simulink model "modello_nave"  (R2023b)
settings: Solver=VariableStepAuto  StartTime=0.0  StopTime=10.0  RelTol=1e-3
values from neighbouring files (symbols this model uses):
  Km1 = 1    [prova_matrici.m]
  Km2 = 1    [prova_matrici.m]
  phi_0 = 0    [prova_matrici.m]
  r_0 = 0    [prova_matrici.m]
  T1 = 1    [prova_matrici.m]
  Tm1 = 1    [prova_matrici.m]
  Tm2 = 1    [prova_matrici.m]
  u_0 = 0    [prova_matrici.m]
  v_0 = 0    [prova_matrici.m]
settings Model: Creator=edoca  LastModifiedBy=jacoc

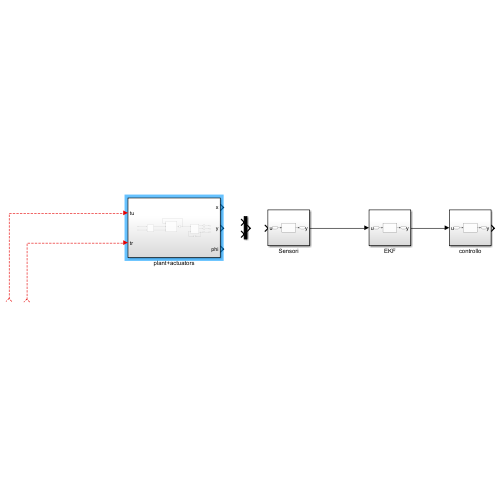
[thumbnail: Simulink's stored preview of the top-level diagram]
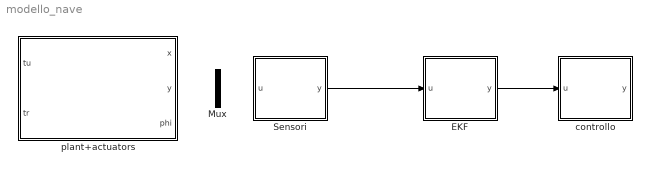
== system modello_nave ==
  EKF : Subsystem
  Mux : Mux  Inputs=2
  Sensori : Subsystem
  controllo : Subsystem
  plant+actuators : Subsystem
  wires:
  ? -> plant+actuators/1(tu)
  ? -> plant+actuators/2(tr)
  EKF/1(y) -> controllo/1(u)
  Sensori/1(y) -> EKF/1(u)

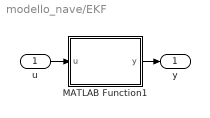
== system modello_nave/EKF ==
  u : Inport
  MATLAB Function1 : MATLAB Function  TreatAsAtomicUnit=on
  y : Outport
  wires:
  u/1 -> MATLAB Function1/1(u)
  MATLAB Function1/1(y) -> y/1

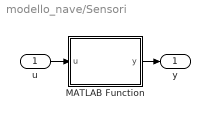
== system modello_nave/Sensori ==
  u : Inport
  MATLAB Function : MATLAB Function  TreatAsAtomicUnit=on
  y : Outport
  wires:
  u/1 -> MATLAB Function/1(u)
  MATLAB Function/1(y) -> y/1

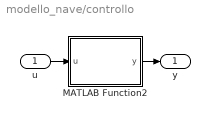
== system modello_nave/controllo ==
  u : Inport
  MATLAB Function2 : MATLAB Function  TreatAsAtomicUnit=on
  y : Outport
  wires:
  u/1 -> MATLAB Function2/1(u)
  MATLAB Function2/1(y) -> y/1

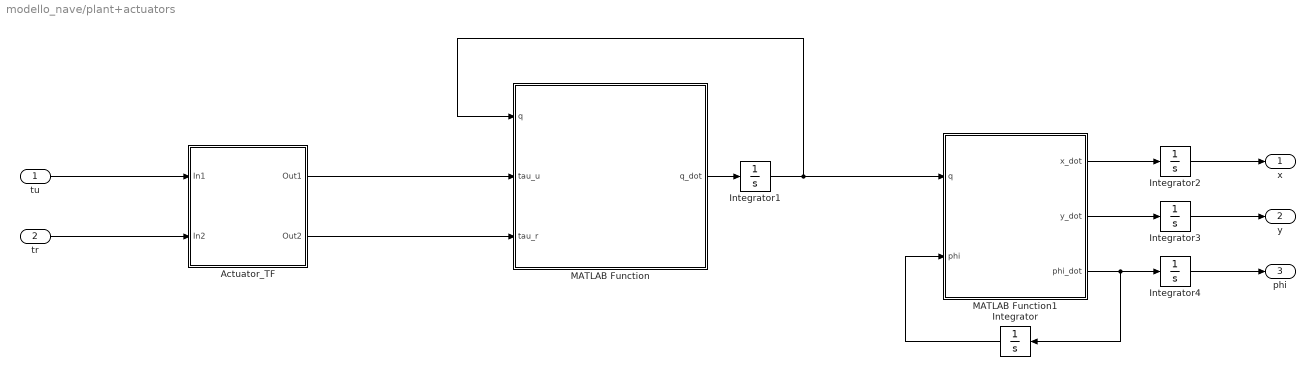
== system modello_nave/plant+actuators ==
  tu : Inport
  tr : Inport  Port=2
  Actuator_TF : Subsystem
  Integrator{,2..4} (4 alike) : Integrator  InitialCondition=phi_0
  Integrator1 : Integrator  InitialCondition=[u_0; v_0; r_0]
  MATLAB Function : MATLAB Function  TreatAsAtomicUnit=on
  MATLAB Function1 : MATLAB Function  TreatAsAtomicUnit=on
  x : Outport
  y : Outport  Port=2
  phi : Outport  Port=3
  wires:
  Integrator1/1 -> MATLAB Function/1(q), MATLAB Function1/1(q)
  MATLAB Function/1(q_dot) -> Integrator1/1
  Integrator/1 -> MATLAB Function1/2(phi)
  MATLAB Function1/3(phi_dot) -> Integrator4/1, Integrator/1
  MATLAB Function1/2(y_dot) -> Integrator3/1
  MATLAB Function1/1(x_dot) -> Integrator2/1
  Integrator2/1 -> x/1
  Integrator3/1 -> y/1
  Integrator4/1 -> phi/1
  tu/1 -> Actuator_TF/1(In1)
  tr/1 -> Actuator_TF/2(In2)
  Actuator_TF/1(Out1) -> MATLAB Function/2(tau_u)
  Actuator_TF/2(Out2) -> MATLAB Function/3(tau_r)

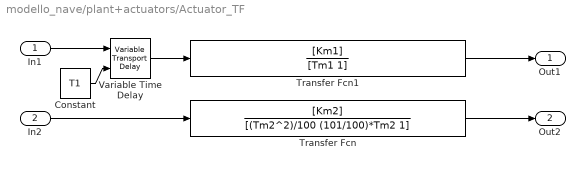
== system modello_nave/plant+actuators/Actuator_TF ==
  In1 : Inport
  In2 : Inport  Port=2
  Constant : Constant  Value=T1
  Transfer Fcn : TransferFcn  Numerator=[Km2]  Denominator=[(Tm2^2)/100 (101/100)*Tm2 1]
  Transfer Fcn1 : TransferFcn  Numerator=[Km1]  Denominator=[Tm1 1]
  Variable Time Delay : VariableTransportDelay  MaximumDelay=100  PadeOrder=1
  Out1 : Outport
  Out2 : Outport  Port=2
  wires:
  Constant/1 -> Variable Time Delay/2
  Variable Time Delay/1 -> Transfer Fcn1/1
  In2/1 -> Transfer Fcn/1
  Transfer Fcn1/1 -> Out1/1
  Transfer Fcn/1 -> Out2/1
  In1/1 -> Variable Time Delay/1

== matlab function modello_nave/plant+actuators/MATLAB Function1 ==
  data: q input; x_dot output; phi input; y_dot output; phi_dot output
function [x_dot, y_dot, phi_dot] = output_dynamic(q, phi)
    
    u = q(1);
    v = q(2);
    r = q(3);

    x_dot = u*cos(phi) - v*sin(phi);
    y_dot = u*sin(phi) + v*cos(phi);
    phi_dot = r;

end

== matlab function modello_nave/plant+actuators/MATLAB Function ==
  data: q input; q_dot output; tau_u input; tau_r input; params parameter
function q_dot  = state_dynamic(q, tau_u, tau_r, params)
    
    m11 = params(1);
    m22 = params(2);
    m33 = params(3);

    d11 = params(4);
    d22 = params(5);
    d33 = params(6);

    u = q(1);
    v = q(2);
    r = q(3);

    % u_dot = (m22/m11)*v*r - (d11/m11)*u + (1/m11)*tau_u;
    % v_dot = -(m11/m22)*u*r - (d22/m22)*v;
    % r_dot = ((m11 - m22)/m33)*u*v - (d33/m33)*r + (1/m33)*tau_r;

    %% Linearization
    % state vector [u, v, r] = q
    
    tau = [tau_u; tau_r];

    A = [-(d11/m11),            (m22/m11)*r,            (m22/m11)*v;
         -(m11/m22)*r,          -(d22/m22),             -(m11/m22)*u;
         ((m11 - m22)/m33)*v,   ((m11 - m22)/m33)*u,    -(d33/m33)];
    
    B = [(1/m11),   0;
            0   ,   0;
            0   ,   (1/m33)];

    q_dot = A*q + B*tau;


    

end

== matlab function modello_nave/Sensori/MATLAB Function ==
  data: u input; y output
function y = fcn(u)

y = u;

== matlab function modello_nave/EKF/MATLAB Function1 ==
  data: u input; y output
function y = fcn(u)

y = u;

== matlab function modello_nave/controllo/MATLAB Function2 ==
  data: u input; y output
function y = fcn(u)

y = u;
